simulink model "Tarea4Sim"  (R2022b)
settings: Solver=ode4  StartTime=0.0  StopTime=10.0  FixedStep=0.001  RelTol=1e-3
values from neighbouring files (symbols this model uses):
  k = 100    [Tarea4SimParameters.m]
  m = 10    [Tarea4SimParameters.m]
  r = 0.05    [Tarea4SimParameters.m]
settings Model: Creator=ferch  LastModifiedBy=ferch

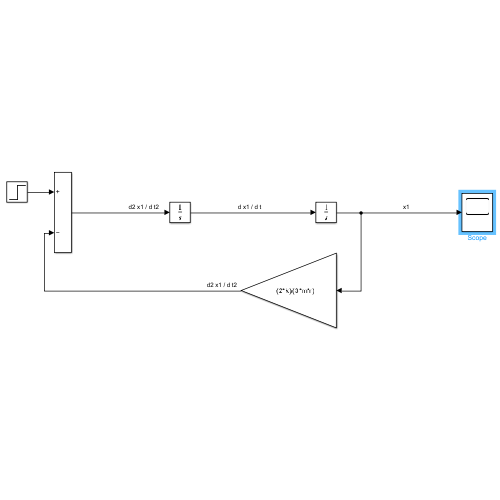
[thumbnail: Simulink's stored preview of the top-level diagram]
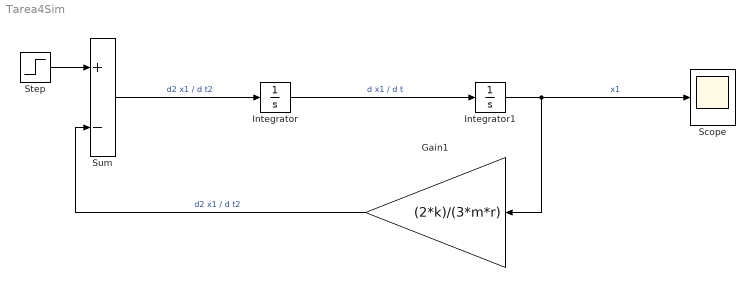
== system Tarea4Sim ==
  Gain1 : Gain  Gain=(2*k)/(3*m*r)
  Integrator : Integrator
  Integrator1 : Integrator  InitialCondition=20*pi/180
  Scope : Scope
  Step : Step  SampleTime=0
  Sum : Sum  Inputs=+-
  wires:
  Integrator/1 -> Integrator1/1  "d x1 / d t"
  Integrator1/1 -> Gain1/1, Scope/1  "x1"
  Sum/1 -> Integrator/1  "d2 x1 / d t2"
  Step/1 -> Sum/1
  Gain1/1 -> Sum/2  "d2 x1 / d t2"
